simulink model "LeeDatosIdentPC"  (R2025a)
settings: Solver=FixedStepDiscrete  StartTime=0.0  StopTime=30  FixedStep=0.01  RelTol=1e-3
undefined symbols (not defined in the file): f
libraries: instrumentlib x1
settings Model: Creator=aj  LastModifiedBy=aj

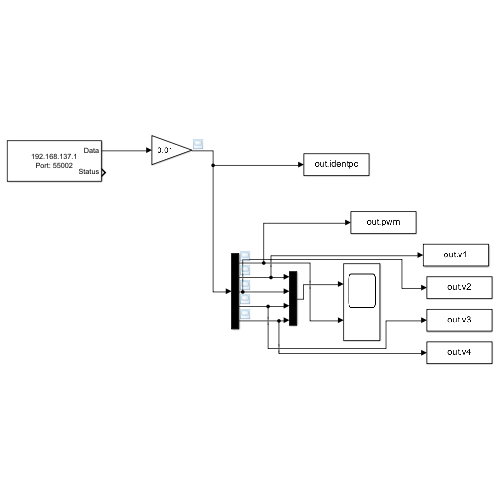
[thumbnail: Simulink's stored preview of the top-level diagram]
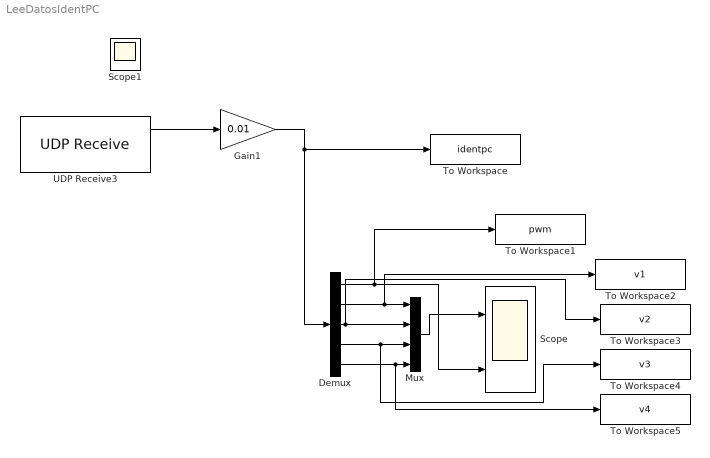
== system LeeDatosIdentPC ==
  Demux : Demux  Outputs=5
  Gain1 : Gain  Gain=0.01  OutDataTypeStr=double
  Mux : Mux
  Scope : Scope  NumInputPorts=2
      settings: ActiveDisplayYMinimum=-0.5275120735168457  ActiveDisplayYMaximum=0.4475102424621582
  To Workspace : ToWorkspace  VariableName=identpc  SampleTime=0.01
      settings: Save2DSignal=2-D array (concatenate along first dimension)
  To Workspace1 : ToWorkspace  VariableName=pwm  SampleTime=0.01
      settings: Save2DSignal=2-D array (concatenate along first dimension)
  To Workspace2 : ToWorkspace  VariableName=v1  SampleTime=0.01
      settings: Save2DSignal=2-D array (concatenate along first dimension)
  To Workspace3 : ToWorkspace  VariableName=v2  SampleTime=0.01
      settings: Save2DSignal=2-D array (concatenate along first dimension)
  To Workspace4 : ToWorkspace  VariableName=v3  SampleTime=0.01
      settings: Save2DSignal=2-D array (concatenate along first dimension)
  To Workspace5 : ToWorkspace  VariableName=v4  SampleTime=0.01
      settings: Save2DSignal=2-D array (concatenate along first dimension)
  UDP Receive3 : instrumentlib/UDP Receive  LocalAddress=192.168.137.1  LocalPort=55002  EnablePortSharing=off  Host=192.168.137.75  Port=55001  GetLatestData=off  DataSize=[ 5, 1 ]  DataType=int16  ASCIIFormatting=%f,  Terminator=LF  CustomTerminator=10  ByteOrder=little-endian  EnableBlockingMode=off  Timeout=10  SampleTime=0.01  SimulateUsing=Interpreted execution
  Scope1 : Scope
  wires:
  UDP Receive3/1 -> Gain1/1
  Demux/1 -> To Workspace1/1, Scope/2
  Demux/2 -> To Workspace2/1, Mux/1
  Demux/4 -> To Workspace4/1, Mux/3
  Mux/1 -> Scope/1
  Demux/5 -> To Workspace5/1, Mux/4
  Gain1/1 -> Demux/1, To Workspace/1
  Demux/3 -> To Workspace3/1, Mux/2
